simulink model "IBC_open_loop2"  (R2021a)
settings: Solver=VariableStepAuto  StartTime=0.0  StopTime=0.02  RelTol=1e-3
InitFcn:
  | Load=2;
  | C=370e-6;
  | L1=1000e-6;
  | L2=1000e-6*(1+normrnd(0,0.05,[1,1]));
  | L3=1000e-6*(1+normrnd(0,0.05,[1,1]));
  | alp=1-0.5;
  | V=2;
libraries: spsCurrentMeasurementLib x11, simulink x10, spsSeriesRLCBranchLib x6, dspsigops x4, spsDiodeLib x3, spsMosfetLib x3, spsDCVoltageSourceLib x2, spsVariableResistorLib x2, spsVoltageMeasurementLib x2, pid_lib x2, spspowerguiLib x2
settings Model: SimulationMode=accelerator  Creator=29721  LastModifiedBy=Dell
settings SolverCC: ZeroCrossAlgorithm=Adaptive  AlgebraicLoopSolver=TrustRegion
settings DebuggingCC: IgnoredZcDiagnostic=none  SFMachineParentedDataDiag=warning

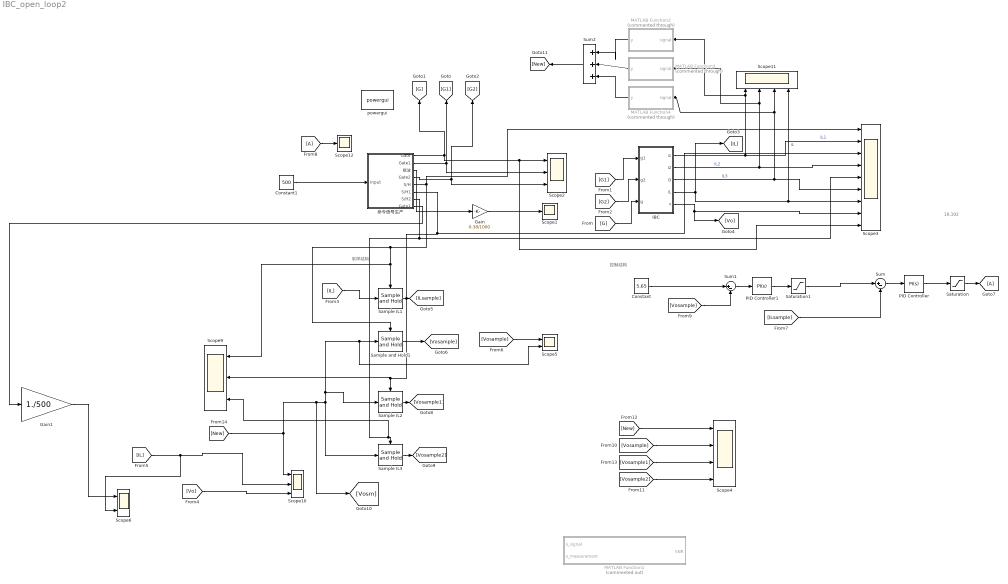
== system IBC_open_loop2 ==
  note: 采样结构
  note: 控制结构
  note: 10.102
  Constant : Constant  Value=5.65
  Constant1 : Constant  Value=500
  Gain : Gain  Gain=0.38/1000
  Gain1 : Gain  Gain=1./500
  IBC : Subsystem  mask{Vin=V, C=C, Load=Load, L1=L1, L2=L1, L3=L1}
  MATLAB Function1 : MATLAB Function  Commented=on  TreatAsAtomicUnit=on
  MATLAB Function2 : MATLAB Function  Commented=through  TreatAsAtomicUnit=on
  MATLAB Function3 : MATLAB Function  Commented=through  TreatAsAtomicUnit=on
  MATLAB Function4 : MATLAB Function  Commented=through  TreatAsAtomicUnit=on
  PID Controller : pid_lib/PID Controller  Controller=PI  Form=Parallel  TimeDomain=Continuous-time  UseExternalTs=off  SampleTime=-1  IntegratorMethod=Forward Euler  FilterMethod=Forward Euler  ControllerParametersSource=internal  P=140  I=186020.6134968  D=0  UseFilter=on  N=100  TunerSelectOption=Transfer Function Based (PID Tuner App)  InitialConditionSource=internal  InitialConditionForIntegrator=0  InitialConditionForFilter=0  DifferentiatorICPrevScaledInput=0  ExternalReset=none  TrackingMode=off  Kt=1  LimitOutput=off  SatLimitsSource=internal  UpperSaturationLimit=inf  LowerSaturationLimit=-inf  LinearizeAsGain=on  AntiWindupMode=none  Kb=1  POutMin=[]  POutMax=[]  IOutMin=[]  IOutMax=[]  DOutMin=[]  DOutMax=[]  NOutMin=[]  NOutMax=[]  SumOutMin=[]  SumOutMax=[]  SaturationOutMin=[]  SaturationOutMax=[]  PParamMin=[]  PParamMax=[]  IParamMin=[]  IParamMax=[]  DParamMin=[]  DParamMax=[]  NParamMin=[]  NParamMax=[]  KbParamMin=[]  KbParamMax=[]  KtParamMin=[]  KtParamMax=[]  KbOutMin=[]  KbOutMax=[]  KtOutMin=[]  KtOutMax=[]  IntegratorOutMin=[]  IntegratorOutMax=[]  FilterOutMin=[]  FilterOutMax=[]  SumI1OutMin=[]  SumI1OutMax=[]  SumI2OutMin=[]  SumI2OutMax=[]  SumI3OutMin=[]  SumI3OutMax=[]  SumI4OutMin=[]  SumI4OutMax=[]  SumDOutMin=[]  SumDOutMax=[]  DifferentiatorOutMin=[]  DifferentiatorOutMax=[]  FilterDiffOutCoefMin=[]  FilterDiffOutCoefMax=[]  ReciprocalOutMin=[]  ReciprocalOutMax=[]  SumDenOutMin=[]  SumDenOutMax=[]  SumNumOutMin=[]  SumNumOutMax=[]  DivideOutMin=[]  DivideOutMax=[]  UdiffTsProdOutMin=[]  UdiffTsProdOutMax=[]  NTsProdOutMin=[]  NTsProdOutMax=[]  UintegralTsProdOutMin=[]  UintegralTsProdOutMax=[]  UngainTsProdOutMin=[]  UngainTsProdOutMax=[]  IntegratorContinuousStateAttributes=''  IntegratorStateMustResolveToSignalObject=off  IntegratorRTWStateStorageClass=Auto  FilterContinuousStateAttributes=''  FilterStateMustResolveToSignalObject=off  FilterRTWStateStorageClass=Auto  ParallelPVariant=InternalParameters  IdealPVariant=Disabled  IVariant=InternalParameters  DVariant=Disabled  IntegratorVariant=Continuous  SatVariant=Disabled  AWVariant=Passthrough  PCopyVariant=Disabled  TRVariant=Disabled  FdbkBlocksVariant=Forward  IdealPFdbkVariant=Disabled  SatFdbkVariant=Disabled  DerivativeFilterVariant=Disabled  NVariant=Disabled  NCopyVariant=Disabled_SignalSpec  FilterICVariant=Disabled  IntegratorICVariant=InternalICs  ExternalResetVariant=Disabled  TRSumVariant=Passthrough  SumFdbkVariant=Disabled  SumVariant=Sum_PI  TsampFilterVariant=InternalTs  TsampNgainVariant=Passthrough  TsampIntegralVariant=Passthrough  ExternalSaturationOutDataTypeStr=Inherit: Same as second input
  PID Controller1 : pid_lib/PID Controller  Controller=PI  Form=Parallel  TimeDomain=Continuous-time  UseExternalTs=off  SampleTime=-1  IntegratorMethod=Forward Euler  FilterMethod=Forward Euler  ControllerParametersSource=internal  P=0.01  I=500  D=0  UseFilter=on  N=100  TunerSelectOption=Transfer Function Based (PID Tuner App)  InitialConditionSource=internal  InitialConditionForIntegrator=0  InitialConditionForFilter=0  DifferentiatorICPrevScaledInput=0  ExternalReset=none  TrackingMode=off  Kt=1  LimitOutput=off  SatLimitsSource=internal  UpperSaturationLimit=inf  LowerSaturationLimit=-inf  LinearizeAsGain=on  AntiWindupMode=none  Kb=1  POutMin=[]  POutMax=[]  IOutMin=[]  IOutMax=[]  DOutMin=[]  DOutMax=[]  NOutMin=[]  NOutMax=[]  SumOutMin=[]  SumOutMax=[]  SaturationOutMin=[]  SaturationOutMax=[]  PParamMin=[]  PParamMax=[]  IParamMin=[]  IParamMax=[]  DParamMin=[]  DParamMax=[]  NParamMin=[]  NParamMax=[]  KbParamMin=[]  KbParamMax=[]  KtParamMin=[]  KtParamMax=[]  KbOutMin=[]  KbOutMax=[]  KtOutMin=[]  KtOutMax=[]  IntegratorOutMin=[]  IntegratorOutMax=[]  FilterOutMin=[]  FilterOutMax=[]  SumI1OutMin=[]  SumI1OutMax=[]  SumI2OutMin=[]  SumI2OutMax=[]  SumI3OutMin=[]  SumI3OutMax=[]  SumI4OutMin=[]  SumI4OutMax=[]  SumDOutMin=[]  SumDOutMax=[]  DifferentiatorOutMin=[]  DifferentiatorOutMax=[]  FilterDiffOutCoefMin=[]  FilterDiffOutCoefMax=[]  ReciprocalOutMin=[]  ReciprocalOutMax=[]  SumDenOutMin=[]  SumDenOutMax=[]  SumNumOutMin=[]  SumNumOutMax=[]  DivideOutMin=[]  DivideOutMax=[]  UdiffTsProdOutMin=[]  UdiffTsProdOutMax=[]  NTsProdOutMin=[]  NTsProdOutMax=[]  UintegralTsProdOutMin=[]  UintegralTsProdOutMax=[]  UngainTsProdOutMin=[]  UngainTsProdOutMax=[]  IntegratorContinuousStateAttributes=''  IntegratorStateMustResolveToSignalObject=off  IntegratorRTWStateStorageClass=Auto  FilterContinuousStateAttributes=''  FilterStateMustResolveToSignalObject=off  FilterRTWStateStorageClass=Auto  ParallelPVariant=InternalParameters  IdealPVariant=Disabled  IVariant=InternalParameters  DVariant=Disabled  IntegratorVariant=Continuous  SatVariant=Disabled  AWVariant=Passthrough  PCopyVariant=Disabled  TRVariant=Disabled  FdbkBlocksVariant=Forward  IdealPFdbkVariant=Disabled  SatFdbkVariant=Disabled  DerivativeFilterVariant=Disabled  NVariant=Disabled  NCopyVariant=Disabled_SignalSpec  FilterICVariant=Disabled  IntegratorICVariant=InternalICs  ExternalResetVariant=Disabled  TRSumVariant=Passthrough  SumFdbkVariant=Disabled  SumVariant=Sum_PI  TsampFilterVariant=InternalTs  TsampNgainVariant=Passthrough  TsampIntegralVariant=Passthrough  ExternalSaturationOutDataTypeStr=Inherit: Same as second input
  Sample IL1 : dspsigops/Sample and Hold  trig=Rising edge  initCond=0  latchinput=off
  Sample IL2 : dspsigops/Sample and Hold  trig=Rising edge  initCond=0  latchinput=off
  Sample IL3 : dspsigops/Sample and Hold  trig=Rising edge  initCond=0  latchinput=off
  Sample and Hold1 : dspsigops/Sample and Hold  trig=Rising edge  initCond=0  latchinput=off
  Saturation : Saturate  UpperLimit=900  LowerLimit=100
  Saturation1 : Saturate  UpperLimit=5  LowerLimit=0
  Scope1 : Scope
  Scope10 : Scope  NumInputPorts=3
  Scope11 : Scope  NumInputPorts=4
  Scope12 : Scope
  Scope2 : Scope  NumInputPorts=3
  Scope3 : Scope  NumInputPorts=9
  Scope4 : Scope  NumInputPorts=4
  Scope5 : Scope  NumInputPorts=2
  Scope6 : Scope  NumInputPorts=2
  Scope9 : Scope  NumInputPorts=3
  Sum : Sum  Inputs=|+-
  Sum1 : Sum  Inputs=|+-
  Sum2 : Sum  Inputs=|+++
  powergui : spspowerguiLib/powergui  Priority=1  SimulationMode=Discrete  SampleTime=2.5e-8  frequency=60  Iterations=50  frequencyindice=0  Pbase=100e6  ErrMax=1e-4  UnitsV=kV  UnitsW=MW  buscounter=0  FunctionMessages=off  echomessages=off  EnableUseOfTLC=off  CurrentSourceSwitches=on  DisableSnubberDevices=off  DisableRonSwitches=off  DisableVfSwitches=off  DisplayEquations=off  AutomaticDiscreteSolvers=on  SolverType=Tustin  Interpol=off  ExternalGateDelay=off  methode=off  Ts=100  x0status=blocks  SPID=off  SwTol=0  HookPort=off  NonlinearTolerance=1e-4  nMaxIteration=100  ContinueOnMaxIteration=off  RestoreLinks=warning  ResistiveCurrentMeasurement=off  Frange=[0:2:500]  Ylog=off  Xlog=on  ShowGrid=off  save=off  variable=ZData  structure=ScopeData  ZoomFFT=off  StartTime=0.033333  cycles=1  DisplayStyle=1  fundamental=300000  FreqAxis=on  MaxFrequency=300000  frequencyindicesteady=1  RmsSteady=1  display=off
  命令信号生产 : Subsystem  mask{Fs=10e3}
      mask prompts: Fs "swicthing frequency"
  wires:
  命令信号生产/1(Gate) -> Scope3/9, Scope2/1, [G]
  命令信号生产/2(Gate1) -> Scope2/2, [G1]
  命令信号生产/4(Gate2) -> Scope2/3, [G2]
  IBC/2(i2) -> Scope3/4, MATLAB Function3/1(signal), Scope11/2  "iL2"
  IBC/5(v) -> Scope3/8, [Vo]
  [G] -> IBC/3(g)
  [G1] -> IBC/1(g1)
  [G2] -> IBC/2(g2)
  Gain/1 -> Scope1/1
  Sum1/1 -> PID Controller1/1
  Constant/1 -> Sum1/1
  [Vosample] -> Sum1/2
  PID Controller/1 -> Saturation/1
  Sum/1 -> PID Controller/1
  [ILsample] -> Sum/2
  Saturation/1 -> [A]
  PID Controller1/1 -> Saturation1/1
  [IL] -> Sample IL1/1
  [Vosample] -> Scope5/1
  Sample IL1/1 -> [ILsample]
  命令信号生产/5(S/H) -> Sample and Hold1/Trigger, Scope9/1, Sample IL1/Trigger, Scope3/1
  Sample and Hold1/1 -> [Vosample]
  Saturation1/1 -> Sum/1
  IBC/1(i1) -> Scope3/2, MATLAB Function2/1(signal), Scope11/1  "iL1"
  Constant1/1 -> 命令信号生产/1(Input)
  IBC/4(iL) -> Scope11/4, Scope3/7, [IL]  "iL"
  Sample IL2/1 -> [Vosample1]
  命令信号生产/3(载波) -> Gain/1
  命令信号生产/7(S/H2) -> Scope9/3, Sample IL3/Trigger, Scope3/5
  [IL] -> Scope6/2, Scope10/2
  Sample IL3/1 -> [Vosample2]
  [Vosample] -> Scope4/2
  [Vosample1] -> Scope4/3
  [Vosample2] -> Scope4/4
  命令信号生产/6(S/H1) -> Scope3/3, Sample IL2/Trigger, Scope9/2
  [New] -> Scope4/1
  IBC/3(i3) -> Scope3/6, Scope11/3, MATLAB Function4/1(signal)  "iL3"
  [New] -> [Vosm], Sample IL3/1, Sample and Hold1/1, Scope5/2, Sample IL2/1, Scope10/1
  [A] -> Scope12/1
  [Vo] -> Scope10/3
  命令信号生产/8(Gate3) -> Gain1/1
  Gain1/1 -> Scope6/1
  MATLAB Function2/1(y) -> Sum2/1
  MATLAB Function3/1(y) -> Sum2/2
  MATLAB Function4/1(y) -> Sum2/3
  Sum2/1 -> [New]

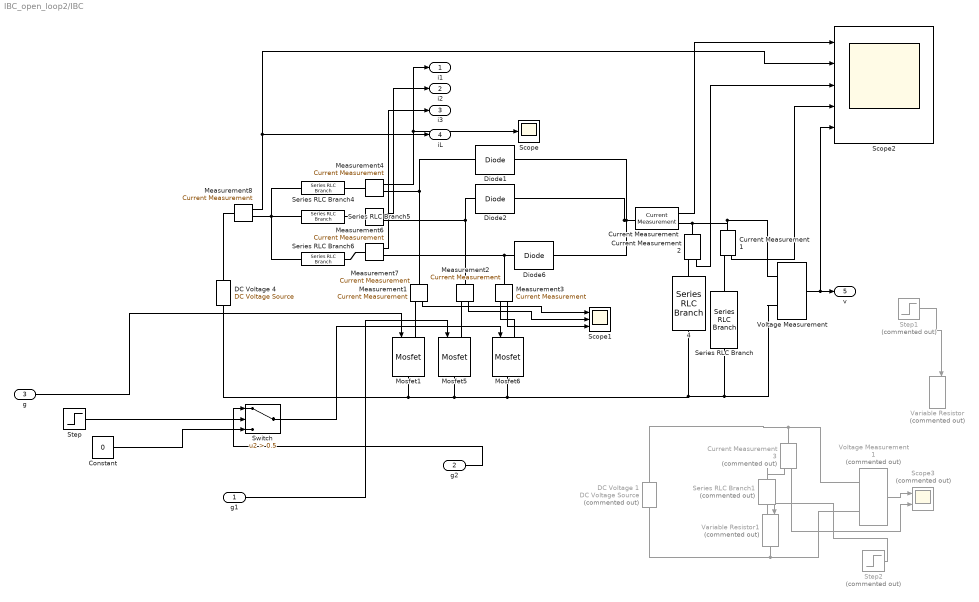
== system IBC_open_loop2/IBC ==
  g1 : Inport
  g2 : Inport  Port=2
  g : Inport  Port=3
  "    4" : spsSeriesRLCBranchLib/Series RLC Branch  LConnTagsString=__new0  RConnTagsString=__new0  BranchType=C  Resistance=0.1  Inductance=69e-3  SetiL0=off  InitialCurrent=0  Capacitance=C  Setx0=off  InitialVoltage=0  Measurements=None
   Measurement{1..4,6..8} (7 alike) : spsCurrentMeasurementLib/Current Measurement  PhasorSimulation=off  OutputType=Complex  PSBequivalent=0
  Constant : Constant  Value=0
  Current Measurement : spsCurrentMeasurementLib/Current Measurement  PhasorSimulation=off  OutputType=Complex  PSBequivalent=0
  Current Measurement1 : spsCurrentMeasurementLib/Current Measurement  PhasorSimulation=off  OutputType=Complex  PSBequivalent=0
  Current Measurement2 : spsCurrentMeasurementLib/Current Measurement  PhasorSimulation=off  OutputType=Complex  PSBequivalent=0
  Current Measurement3 : spsCurrentMeasurementLib/Current Measurement  Commented=on  PhasorSimulation=off  OutputType=Complex  PSBequivalent=0
  DC Voltage 1 : spsDCVoltageSourceLib/DC Voltage Source  Commented=on  Amplitude=Vin  Measurements=Voltage
  DC Voltage 4 : spsDCVoltageSourceLib/DC Voltage Source  Amplitude=Vin  Measurements=Voltage
  Diode1 : spsDiodeLib/Diode  Ron=0.001  Lon=0  Vf=0.8  IC=0  UseSnubber=off  Rs=inf  Cs=250e-9  Measurements=off
  Diode2 : spsDiodeLib/Diode  Ron=0.001  Lon=0  Vf=0.8  IC=0  UseSnubber=off  Rs=inf  Cs=250e-9  Measurements=off
  Diode6 : spsDiodeLib/Diode  Ron=0.001  Lon=0  Vf=0.8  IC=0  UseSnubber=off  Rs=inf  Cs=250e-9  Measurements=off
  Mosfet1 : spsMosfetLib/Mosfet  Ron=0.1  Lon=0  Rd=0.01  Vfd=0  IC=0  Rs=1e5  Cs=inf  Measurements=off
  Mosfet5 : spsMosfetLib/Mosfet  Ron=0.1  Lon=0  Rd=0.01  Vfd=0  IC=0  Rs=1e5  Cs=inf  Measurements=off
  Mosfet6 : spsMosfetLib/Mosfet  Ron=0.1  Lon=0  Rd=0.01  Vfd=0  IC=0  Rs=1e5  Cs=inf  Measurements=off
  Scope : Scope
  Scope1 : Scope  NumInputPorts=3
  Scope2 : Scope  NumInputPorts=5
  Scope3 : Scope  Commented=on  NumInputPorts=2
  Series RLC Branch : spsSeriesRLCBranchLib/Series RLC Branch  LConnTagsString=__new0  RConnTagsString=__new0  BranchType=R  Resistance=2  Inductance=1e-3  SetiL0=off  InitialCurrent=0  Capacitance=1e-6  Setx0=off  InitialVoltage=0  Measurements=None
  Series RLC Branch1 : spsSeriesRLCBranchLib/Series RLC Branch  Commented=on  LConnTagsString=__new0  RConnTagsString=__new0  BranchType=R  Resistance=0.0001  Inductance=1e-3  SetiL0=off  InitialCurrent=0  Capacitance=1e-6  Setx0=off  InitialVoltage=0  Measurements=None
  Series RLC Branch4 : spsSeriesRLCBranchLib/Series RLC Branch  LConnTagsString=__new0  RConnTagsString=__new0  BranchType=L  Resistance=0  Inductance=L1  SetiL0=off  InitialCurrent=0  Capacitance=1e-6  Setx0=off  InitialVoltage=0  Measurements=None
  Series RLC Branch5 : spsSeriesRLCBranchLib/Series RLC Branch  LConnTagsString=__new0  RConnTagsString=__new0  BranchType=L  Resistance=0  Inductance=L2  SetiL0=off  InitialCurrent=0  Capacitance=1e-6  Setx0=off  InitialVoltage=0  Measurements=None
  Series RLC Branch6 : spsSeriesRLCBranchLib/Series RLC Branch  LConnTagsString=__new0  RConnTagsString=__new0  BranchType=L  Resistance=0  Inductance=L3  SetiL0=off  InitialCurrent=0  Capacitance=1e-6  Setx0=off  InitialVoltage=0  Measurements=None
  Step : Step  Time=0.01  Before=1  After=0  SampleTime=0
  Step1 : Step  Commented=on  Time=0.009  Before=1  After=2  SampleTime=0
  Step2 : Step  Commented=on  Time=0.008  Before=1  After=2  SampleTime=0
  Switch : Switch  Criteria=u2 > Threshold  Threshold=0.5
  Variable Resistor : spsVariableResistorLib/Variable Resistor  Commented=on  Rabsmin=1e-3
      settings: SourceProductBaseCode=PS
  Variable Resistor1 : spsVariableResistorLib/Variable Resistor  Commented=on  Rabsmin=1e-3
      settings: SourceProductBaseCode=PS
  Voltage Measurement : spsVoltageMeasurementLib/Voltage Measurement  PhasorSimulation=off  OutputType=Complex  PSBequivalent=0
  Voltage Measurement1 : spsVoltageMeasurementLib/Voltage Measurement  Commented=on  PhasorSimulation=off  OutputType=Complex  PSBequivalent=0
  i1 : Outport
  i2 : Outport  Port=2
  i3 : Outport  Port=3
  iL : Outport  Port=4
  v : Outport  Port=5
  wires:
  g2/1 -> Switch/1
  " Measurement4"/1 -> Scope/1, i1/1
  " Measurement6"/1 -> i2/1
  Voltage Measurement/1 -> Scope2/5, v/1
  " Measurement7"/1 -> i3/1
  Step/1 -> Switch/2
  " Measurement1"/1 -> Scope1/1
  " Measurement2"/1 -> Scope1/2
  g/1 -> Mosfet1/1
  Constant/1 -> Switch/3
  g1/1 -> Mosfet5/1
  " Measurement3"/1 -> Scope1/3
  Switch/1 -> Mosfet6/1
  " Measurement8"/1 -> Scope2/2, iL/1
  Step1/1 -> Variable Resistor/1
  Current Measurement/1 -> Scope2/1
  Current Measurement1/1 -> Scope2/4
  Current Measurement2/1 -> Scope2/3
  Step2/1 -> Variable Resistor1/1
  Voltage Measurement1/1 -> Scope3/1
  Current Measurement3/1 -> Scope3/2
  connections:
  Diode6/LConn1 -- " Measurement7"/RConn1 -- " Measurement3"/LConn1
  Diode2/LConn1 -- " Measurement2"/LConn1 -- " Measurement6"/RConn1
  " Measurement8"/LConn1 -- DC Voltage 4/RConn1
  Mosfet5/RConn1 -- Mosfet6/RConn1 -- Voltage Measurement/LConn2 -- Series RLC Branch/RConn1 -- "    4"/RConn1 -- Mosfet1/RConn1 -- DC Voltage 4/LConn1
  Series RLC Branch4/LConn1 -- Series RLC Branch5/LConn1 -- Series RLC Branch6/LConn1 -- " Measurement8"/RConn1
  " Measurement4"/LConn1 -- Series RLC Branch4/RConn1
  " Measurement6"/LConn1 -- Series RLC Branch5/RConn1
  " Measurement7"/LConn1 -- Series RLC Branch6/RConn1
  Diode6/RConn1 -- Current Measurement/LConn1 -- Diode2/RConn1 -- Diode1/RConn1
  " Measurement4"/RConn1 -- " Measurement1"/LConn1 -- Diode1/LConn1
  " Measurement1"/RConn1 -- Mosfet1/LConn1
  " Measurement2"/RConn1 -- Mosfet5/LConn1
  " Measurement3"/RConn1 -- Mosfet6/LConn1
  Voltage Measurement/LConn1 -- Current Measurement2/LConn1 -- Current Measurement/RConn1 -- Current Measurement1/LConn1
  Current Measurement1/RConn1 -- Series RLC Branch/LConn1
  Current Measurement2/RConn1 -- "    4"/LConn1
  Voltage Measurement1/LConn1 -- DC Voltage 1/RConn1 -- Current Measurement3/LConn1
  DC Voltage 1/LConn1 -- Voltage Measurement1/LConn2 -- Variable Resistor1/RConn1
  Series RLC Branch1/RConn1 -- Variable Resistor1/LConn1
  Series RLC Branch1/LConn1 -- Current Measurement3/RConn1

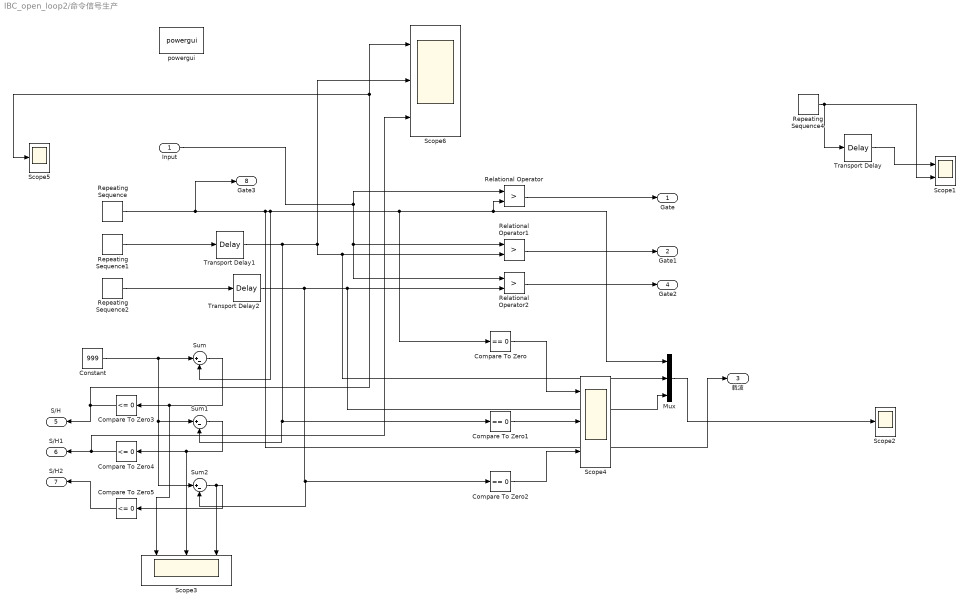
== system IBC_open_loop2/命令信号生产 ==
  Input : Inport
  Compare To Zero : simulink/Logic and Bit Operations/Compare To Zero  relop===  OutDataTypeStr=boolean
  Compare To Zero1 : simulink/Logic and Bit Operations/Compare To Zero  relop===  OutDataTypeStr=boolean
  Compare To Zero2 : simulink/Logic and Bit Operations/Compare To Zero  relop===  OutDataTypeStr=boolean
  Compare To Zero3 : simulink/Logic and Bit Operations/Compare To Zero  relop=<=  OutDataTypeStr=boolean
  Compare To Zero4 : simulink/Logic and Bit Operations/Compare To Zero  relop=<=  OutDataTypeStr=boolean
  Compare To Zero5 : simulink/Logic and Bit Operations/Compare To Zero  relop=<=  OutDataTypeStr=boolean
  Constant : Constant  Value=999
  Mux : Mux  Inputs=3
  Relational Operator : RelationalOperator  Operator=>  OutDataTypeStr=boolean  RndMeth=Simplest
  Relational Operator1 : RelationalOperator  Operator=>  OutDataTypeStr=boolean  RndMeth=Simplest
  Relational Operator2 : RelationalOperator  Operator=>  OutDataTypeStr=boolean  RndMeth=Simplest
  Repeating Sequence : simulink/Sources/Repeating Sequence  rep_seq_t=[0 1./Fs./2 1./Fs]  rep_seq_y=[0 1000 0]
  Repeating Sequence1 : simulink/Sources/Repeating Sequence  rep_seq_t=[1./Fs./3 5./Fs./6 4./Fs./3]  rep_seq_y=[0 1000 0]
  Repeating Sequence2 : simulink/Sources/Repeating Sequence  rep_seq_t=[2./Fs./3 7./Fs./6 5./Fs./3]  rep_seq_y=[0 1000 0]
  Repeating Sequence4 : simulink/Sources/Repeating Sequence  rep_seq_t=[0 1./100e3./2 1./100e3]  rep_seq_y=[0 1000 0]
  Scope1 : Scope  NumInputPorts=2
  Scope2 : Scope
  Scope3 : Scope  NumInputPorts=3
  Scope4 : Scope  NumInputPorts=3
  Scope5 : Scope
  Scope6 : Scope  NumInputPorts=3
  Sum : Sum  Inputs=|+-
  Sum1 : Sum  Inputs=|+-
  Sum2 : Sum  Inputs=|+-
  Transport Delay : TransportDelay  DelayTime=1./100e3./3
  Transport Delay1 : TransportDelay  DelayTime=1./Fs./3
  Transport Delay2 : TransportDelay  DelayTime=2./Fs./3
  powergui : spspowerguiLib/powergui  Priority=1  SimulationMode=Discrete  SampleTime=2.5e-8  frequency=60  Iterations=50  frequencyindice=0  Pbase=100e6  ErrMax=1e-4  UnitsV=kV  UnitsW=MW  buscounter=0  FunctionMessages=off  echomessages=off  EnableUseOfTLC=off  CurrentSourceSwitches=on  DisableSnubberDevices=off  DisableRonSwitches=off  DisableVfSwitches=off  DisplayEquations=off  AutomaticDiscreteSolvers=off  SolverType=Tustin  Interpol=off  ExternalGateDelay=off  methode=off  Ts=100  x0status=blocks  SPID=off  SwTol=0  HookPort=off  NonlinearTolerance=1e-4  nMaxIteration=100  ContinueOnMaxIteration=off  RestoreLinks=warning  ResistiveCurrentMeasurement=off  Frange=[0:2:500]  Ylog=off  Xlog=on  ShowGrid=off  save=off  variable=ZData  structure=ScopeData  ZoomFFT=off  StartTime=0.033333  cycles=1  DisplayStyle=1  fundamental=300000  FreqAxis=on  MaxFrequency=300000  frequencyindicesteady=1  RmsSteady=1  display=off
  Gate : Outport
  Gate1 : Outport  Port=2
  载波 : Outport  Port=3
  Gate2 : Outport  Port=4
  S/H : Outport  Port=5
  S/H1 : Outport  Port=6
  S/H2 : Outport  Port=7
  Gate3 : Outport  Port=8
  wires:
  Input/1 -> Relational Operator1/1, Relational Operator2/1, Relational Operator/1
  Compare To Zero/1 -> Scope4/1
  Relational Operator/1 -> Gate/1
  Repeating Sequence1/1 -> Transport Delay1/1
  Relational Operator1/1 -> Gate1/1
  Repeating Sequence2/1 -> Transport Delay2/1
  Repeating Sequence/1 -> Gate3/1, Mux/1, Relational Operator/2, Compare To Zero/1, Sum/2, 载波/1
  Relational Operator2/1 -> Gate2/1
  Repeating Sequence4/1 -> Transport Delay/1, Scope1/2
  Transport Delay/1 -> Scope1/1
  Mux/1 -> Scope2/1
  Transport Delay1/1 -> Sum1/2, Compare To Zero1/1, Scope6/2, Mux/2, Relational Operator1/2
  Compare To Zero1/1 -> Scope4/2
  Compare To Zero2/1 -> Scope4/3
  Sum/1 -> Scope3/1, Compare To Zero3/1
  Sum1/1 -> Compare To Zero4/1, Scope3/2
  Transport Delay2/1 -> Sum2/2, Compare To Zero2/1, Mux/3, Relational Operator2/2
  Sum2/1 -> Scope3/3, Compare To Zero5/1
  Constant/1 -> Sum2/1, Sum1/1, Sum/1
  Compare To Zero3/1 -> Scope6/1, Scope5/1, S/H/1
  Compare To Zero4/1 -> Scope6/3, S/H1/1
  Compare To Zero5/1 -> S/H2/1

== matlab function IBC_open_loop2/MATLAB Function2 ==
  data: signal input; y output
function y    = Add_Noise(signal)
%================== Add the noise to the outputvoltage===================%
x_signal = signal;
% Estimate the power of input signal
Ps = sum(x_signal.^2)./length(x_signal);
% Calculate the power of noise
SNR = 50;
Pn = Ps/(10^(SNR/10));
% Generate the noise
Noise = sqrt(Pn).*randn(length(x_signal),1);
A_signal = sqrt(sum(x_signal.^2)/(length(x_signal)));
A_noise  = sqrt(sum(Noise.^2)/(length(Noise)));
SNR1 = 20*log10(A_signal/A_noise);
x_measurement = x_signal+Noise;
y = x_measurement;

== matlab function IBC_open_loop2/MATLAB Function3 ==
  data: signal input; y output
function y    = Add_Noise(signal)
%================== Add the noise to the outputvoltage===================%
x_signal = signal;
% Estimate the power of input signal
Ps = sum(x_signal.^2)./length(x_signal);
% Calculate the power of noise
SNR = 60;
Pn = Ps/(10^(SNR/10));
% Generate the noise
Noise = sqrt(Pn).*randn(length(x_signal),1);
A_signal = sqrt(sum(x_signal.^2)/(length(x_signal)));
A_noise  = sqrt(sum(Noise.^2)/(length(Noise)));
SNR1 = 20*log10(A_signal/A_noise);
x_measurement = x_signal+Noise;
y = x_measurement;

== matlab function IBC_open_loop2/MATLAB Function4 ==
  data: signal input; y output
function y    = Add_Noise(signal)
%================== Add the noise to the outputvoltage===================%
x_signal = signal;
% Estimate the power of input signal
Ps = sum(x_signal.^2)./length(x_signal);
% Calculate the power of noise
SNR = 60;
Pn = Ps/(10^(SNR/10));
% Generate the noise
Noise = sqrt(Pn).*randn(length(x_signal),1);
A_signal = sqrt(sum(x_signal.^2)/(length(x_signal)));
A_noise  = sqrt(sum(Noise.^2)/(length(Noise)));
SNR1 = 20*log10(A_signal/A_noise);
x_measurement = x_signal+Noise;
y = x_measurement;

== matlab function IBC_open_loop2/MATLAB Function1 ==
  data: x_signal input; SNR output; x_measurement input
function SNR = SNR_calculte(x_signal,x_measurement)
%================== Calculate the SNR ===================%
x_noise = x_measurement-x_signal;
% Calculate the power of the signal and noise
Ps = sum(x_signal.^2)./length(x_signal);
Pn = sum(x_noise.^2)./length(x_noise);
% Calculate the SNR
SNR = 10*log10(Ps/Pn);
